simulink model "counter"  (R2015a)
settings: Solver=ode45  StartTime=0.0  StopTime=10.0  RelTol=1e-3
InitFcn:
  | %% DSPBuilder Start
  | alt_dspbuilder_update_model(bdroot)
  | %% DSPBuilder End
libraries: allblocks_alteradspbuilder2 x13
settings Model: Creator=ASUS  LastModifiedBy=ASUS

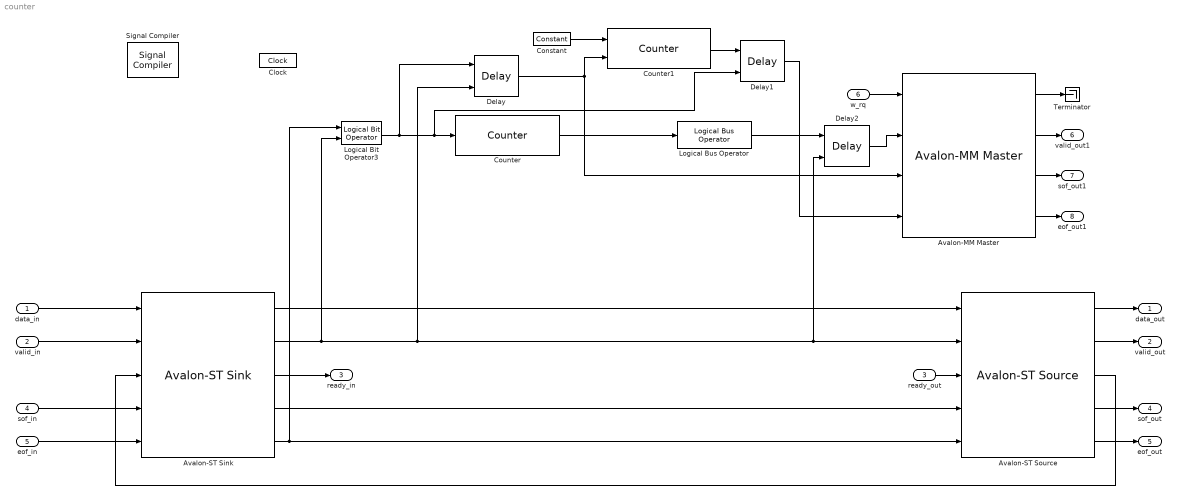
== system counter ==
  data_in : Inport
  valid_in : Inport  Port=2
  "ready_out " : Inport  Port=3
  sof_in : Inport  Port=4
  eof_in : Inport  Port=5
  w_rq : Inport  Port=6
  Avalon-MM Master : allblocks_alteradspbuilder2/Avalon-MM Master  iofile=C:\Users\ASUS\Desktop\final_sift_fpga\tb_gauss\gauss_Avalon-MM+Master_waitrequest.salt,C:\Users\ASUS\Desktop\final_sift_fpga\tb_gauss\gauss_Avalon-MM+Master_address.capture,C:\Users\ASUS\Desktop\final_sift_fpga\tb_gauss\gauss_Avalon-MM+Master_write.capture,C:\Users\ASUS\Desktop\final_sift_fpga\tb_gauss\gauss_Avalon-MM+Master_writedata.capture,  SpecifyClock=off  addrWidth=32  addrType=Write  BusType=Unsigned Integer  bwl=32  bwr=0  byteEnable=off  flowCtrl=off  pipeline=off  flush=off  burst=off  maxBurst=4  irq=off  irq_mode=Prioritized  externalType=Inferred  PORTTYPE=Input
  Avalon-ST Sink : allblocks_alteradspbuilder2/Avalon-ST Sink  iofile=C:\Users\ASUS\Desktop\final_sift_fpga\tb_gauss\gauss_Avalon-ST+Sink_data.salt,C:\Users\ASUS\Desktop\final_sift_fpga\tb_gauss\gauss_Avalon-ST+Sink_valid.salt,C:\Users\ASUS\Desktop\final_sift_fpga\tb_gauss\gauss_Avalon-ST+Sink_ready.capture,C:\Users\ASUS\Desktop\final_sift_fpga\tb_gauss\gauss_Avalon-ST+Sink_startofpacket.salt,C:\Users\ASUS\Desktop\final_sift_fpga\tb_gauss\gauss_Avalon-ST+Sink_endofpacket.salt,  SpecifyClock=off  BusType=Unsigned Integer  bwl=24  bwr=0  symbolWidth=8  symbolsPerBeat=3  numOfChannels=0  numOfErrorDescriptors=0  endOfPacket=on  startOfPacket=on  empty=off  readyLatency=1  externalType=Inferred  PORTTYPE=Output
  Avalon-ST Source : allblocks_alteradspbuilder2/Avalon-ST Source  iofile=C:\Users\ASUS\Desktop\final_sift_fpga\tb_gauss\gauss_Avalon-ST+Source_data.capture,C:\Users\ASUS\Desktop\final_sift_fpga\tb_gauss\gauss_Avalon-ST+Source_valid.capture,C:\Users\ASUS\Desktop\final_sift_fpga\tb_gauss\gauss_Avalon-ST+Source_ready.salt,C:\Users\ASUS\Desktop\final_sift_fpga\tb_gauss\gauss_Avalon-ST+Source_startofpacket.capture,C:\Users\ASUS\Desktop\final_sift_fpga\tb_gauss\gauss_Avalon-ST+Source_endofpacket.capture,  SpecifyClock=off  BusType=Unsigned Integer  bwl=24  bwr=0  symbolWidth=8  symbolsPerBeat=3  numOfChannels=0  numOfErrorDescriptors=0  endOfPacket=on  startOfPacket=on  empty=off  readyLatency=1  externalType=Inferred  PORTTYPE=Input
  Clock : allblocks_alteradspbuilder2/Clock  ClockPeriod=10/1.5  ClockPeriodUnit=ns  SampleTime=1  ResetLatency=0  ResetRegisterCascadeDepth=0  SimulationStartCycle=5  PhaseOffset=0  Reset=aclr  ResetType=Active Low  Export=off
  Constant : allblocks_alteradspbuilder2/Constant  mask_cst=1  BusType=Single Bit  bwl=8  bwr=0  roundMode=Truncate  satMode=Wrap  SpecifyClock=off  allowFloatingPointOverride=on  logOutputs=off  logFile=C:\Users\ASUS\Desktop\final_sift_fpga\tb_gauss\gauss_Constant.fixedpointlog
  Counter : allblocks_alteradspbuilder2/Counter  BusType=Unsigned Integer  bwl=25  bwr=0  use_modulo=on  modulo=640*480  SpecifyClock=off  direction=Increment  use_sload=off  use_sset=off  svalue=1  use_clk_ena=off  use_ena=on  use_sclr=off  pipeline_display=1
  Counter1 : allblocks_alteradspbuilder2/Counter  BusType=Unsigned Integer  bwl=25  bwr=0  use_modulo=on  modulo=10000000  SpecifyClock=off  direction=Increment  use_sload=off  use_sset=off  svalue=1  use_clk_ena=off  use_ena=on  use_sclr=on  pipeline_display=1
  Delay : allblocks_alteradspbuilder2/Delay  pipeline=5  pipeline_display=5  ClockPhase=1  use_ena=on  use_sclr=off  allowFloatingPointOverride=on  logOutputs=off  logFile=C:\Users\ASUS\Desktop\final_sift_fpga\tb_gauss\gauss_Delay.fixedpointlog  use_init=off  reset_value=1
  Delay1 : allblocks_alteradspbuilder2/Delay  pipeline=1  pipeline_display=1  ClockPhase=1  use_ena=on  use_sclr=off  allowFloatingPointOverride=on  logOutputs=off  logFile=C:\Users\ASUS\Desktop\final_sift_fpga\tb_gauss\gauss_Delay1.fixedpointlog  use_init=off  reset_value=1
  Delay2 : allblocks_alteradspbuilder2/Delay  pipeline=5  pipeline_display=5  ClockPhase=1  use_ena=on  use_sclr=off  allowFloatingPointOverride=on  logOutputs=off  logFile=C:\Users\ASUS\Desktop\final_sift_fpga\tb_gauss\gauss_Delay2.fixedpointlog  use_init=off  reset_value=1
  Logical Bit Operator3 : allblocks_alteradspbuilder2/Logical Bit Operator  LogicalOperator=AND  user_inputs=2  pipeline_display=0
  Logical Bus Operator : allblocks_alteradspbuilder2/Logical Bus Operator  BusType=Unsigned Integer  bwl=25  bwr=0  LogicalOp_text=Shift Left  mask_value_num=-5  shift_amount=2  force_sign_ext=on  pipeline_display=0
  Signal Compiler : allblocks_alteradspbuilder2/Signal Compiler  DeviceFamily=Cyclone IV GX  DisableEarlyHDLGeneration=off  EnableSignalTap=off  SignalTapDepth=128  UseBoardBlock=off  StpUseDefaultClock=on  StpClock=Clock  ExportDir=C:\altera\16.0\quartus\dsp_builder  MAX10_ProgrammingMode=Internal Flash (SDM) Single Boot
  Terminator : Terminator
  data_out : Outport
  valid_out : Outport  Port=2
  "ready_in " : Outport  Port=3
  sof_out : Outport  Port=4
  eof_out : Outport  Port=5
  valid_out1 : Outport  Port=6
  sof_out1 : Outport  Port=7
  eof_out1 : Outport  Port=8
  wires:
  data_in/1 -> Avalon-ST Sink/1
  valid_in/1 -> Avalon-ST Sink/2
  sof_in/1 -> Avalon-ST Sink/4
  eof_in/1 -> Avalon-ST Sink/5
  Avalon-ST Source/1 -> data_out/1
  Avalon-ST Source/2 -> valid_out/1
  Avalon-ST Source/4 -> sof_out/1
  Avalon-ST Source/5 -> eof_out/1
  Avalon-ST Sink/4 -> Avalon-ST Source/4
  Avalon-ST Sink/5 -> Logical Bit Operator3/1, Avalon-ST Source/5
  Avalon-ST Source/3 -> Avalon-ST Sink/3
  Avalon-ST Sink/3 -> "ready_in "/1
  "ready_out "/1 -> Avalon-ST Source/3
  Avalon-ST Sink/1 -> Avalon-ST Source/1
  w_rq/1 -> Avalon-MM Master/1
  Avalon-MM Master/1 -> Terminator/1
  Avalon-MM Master/2 -> valid_out1/1
  Avalon-MM Master/3 -> sof_out1/1
  Avalon-MM Master/4 -> eof_out1/1
  Counter/1 -> Logical Bus Operator/1
  Logical Bus Operator/1 -> Delay2/1
  Logical Bit Operator3/1 -> Delay1/2, Counter/1, Delay/1
  Counter1/1 -> Delay1/1
  Constant/1 -> Counter1/1
  Delay/1 -> Counter1/2, Avalon-MM Master/3
  Delay1/1 -> Avalon-MM Master/4
  Avalon-ST Sink/2 -> Logical Bit Operator3/2, Delay/2, Delay2/2, Avalon-ST Source/2
  Delay2/1 -> Avalon-MM Master/2
